simulink model "receiver1"  (R2025a)
settings: Solver=FixedStepAuto  StartTime=0.0  StopTime=10.0  RelTol=1e-3
undefined symbols (not defined in the file): q
libraries: androiduilib x3, dspxfrm3 x2, androidaudiovideolib x1, androidcommunicationlib x1
settings Model: Creator=sahas  LastModifiedBy=sahas
settings OptimizationCC: DefaultParameterBehavior=Inlined  EnhancedBackFolding=on  PassReuseOutputArgsAs=Individual arguments  ZeroExternalMemoryAtStartup=off  ZeroInternalMemoryAtStartup=off  MaxStackSize=64  OptimizeBlockOrder=speed  DifferentSizesBufferReuse=on  OptimizationCustomize=off  EfficientTunableParamExpr=on
settings DebuggingCC: ParameterTunabilityLossMsg=error
settings HardwareCC: ProdBitPerLong=64.0  ProdLargestAtomicInteger=LongLong  ProdLargestAtomicFloat=Double  ProdLongLongMode=on  ProdHWDeviceType=ARM Compatible->ARM Cortex-A (64-bit)  UseEmbeddedCoderFeatures=off
settings SFSimCC: MATLABDynamicMemAlloc=off
settings RTWCC: SystemTargetFile=ert.tlc  HardwareBoard=Android Device (64bit)  TLCOptions="-aInlineSetEventsForThisBaseRateFcn=TLC_FALSE -aSuppressMultiTaskScheduler=TLC_FALSE  -aRateBasedStepFcn=0"  TemplateMakefile=ert_default_tmf  RTWVerbose=off  Toolchain=Android SDK/NDK Tools  Description=Embedded Coder
settings CodeAppCC: ForceParamTrailComments=on  IgnoreCustomStorageClasses=off  OperatorAnnotations=on  SimulinkDataObjDesc=on  SFDataObjDesc=on  InsertBlockDesc=on
settings ERTTargetCC: ExtModeTransport=0.0  ExtModeStaticAlloc=off  ExtModeMexFile=ext_comm  ExtModeIntrfLevel=Level1  SupportNonInlinedSFcns=on

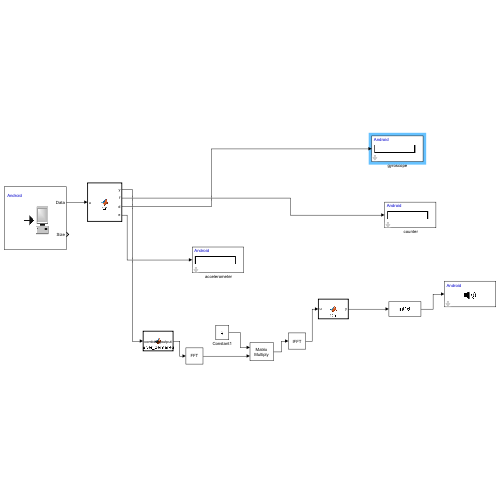
[thumbnail: Simulink's stored preview of the top-level diagram]
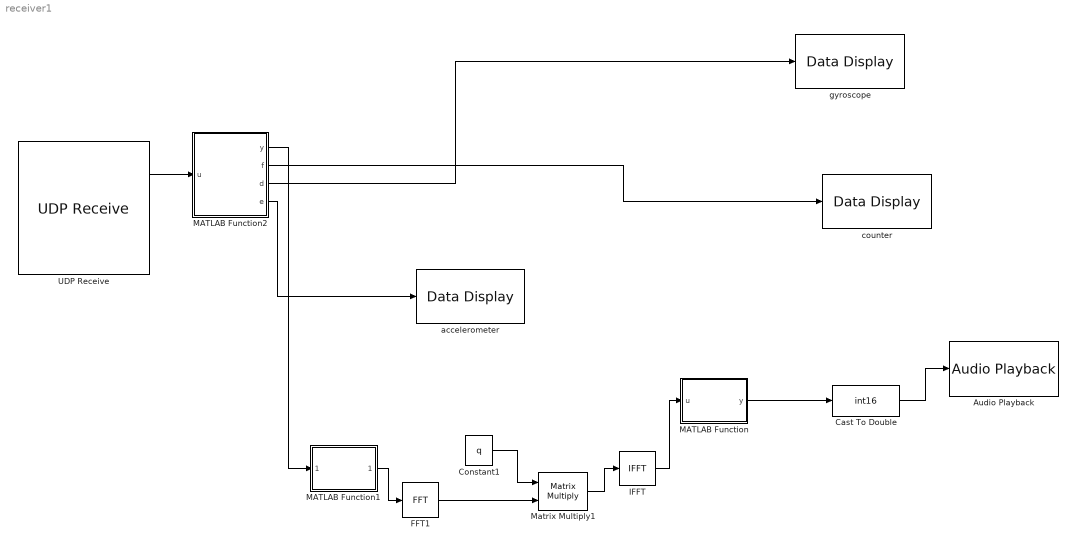
== system receiver1 ==
  " accelerometer" : androiduilib/Data Display  DataDisplayId=receiver1/_accelerometer  Format=Float  Precision=6  SimulateUsing=Code generation  blockPlatform=Android
  " counter" : androiduilib/Data Display  DataDisplayId=receiver1/_counter  Format=Float  Precision=6  SimulateUsing=Code generation  blockPlatform=Android
  Audio Playback : androidaudiovideolib/Audio Playback  SampleFreq=16000  AudioSamplingFreq=16000  SampleTime=0.1  DeviceStr=0  QueueDuration=0  BlockPlatform=Android
  Cast To Double : DataTypeConversion  OutDataTypeStr=int16  SaturateOnIntegerOverflow=off  RndMeth=Floor
  Constant1 : Constant  Value=q  VectorParams1D=off
  FFT1 : dspxfrm3/FFT  FFTImplementation=Auto  CompMethod=Table lookup  TableOpt=NEW  TableOptActive=Speed  BitRevOrder=off  Normalize=off  InheritFFTLength=on  FFTLength=64  WrapInput=on  roundingMode=Ceiling  overflowMode=off  firstCoeffDataTypeStr=Inherit: Same word length as input  firstCoeffLastDataTypeStr=Inherit: Same word length as input  outputMin=[]  outputMax=[]
  IFFT : dspxfrm3/IFFT  FFTImplementation=Auto  CompMethod=Table lookup  TableOpt=NEW  TableOptActive=Speed  BitRevOrder=off  cs_in=off  Normalize=on  InheritFFTLength=on  FFTLength=64  WrapInput=on  mode=Real  outSamplingMode=Sample based  roundingMode=Ceiling  overflowMode=off  firstCoeffDataTypeStr=Inherit: Same word length as input  firstCoeffLastDataTypeStr=Inherit: Same word length as input  outputMin=[]  outputMax=[]
  MATLAB Function : MATLAB Function  TreatAsAtomicUnit=on
  MATLAB Function1 : MATLAB Function  TreatAsAtomicUnit=on
  MATLAB Function2 : MATLAB Function  TreatAsAtomicUnit=on
  Matrix Multiply1 : Product  Multiplication=Matrix(*)
  UDP Receive : androidcommunicationlib/UDP Receive  localURL='0.0.0.0'  localPort=28000  remoteURL='0.0.0.0'  remotePort=-1  recvBufferSize=8192  signalDatatype=double  dims=1031  isVarSize=off  showBlockingTime=off  blockingTime=0  sampletime=0.016  blockPlatform=Android
  gyroscope : androiduilib/Data Display  DataDisplayId=receiver1/gyroscope  Format=Float  Precision=6  SimulateUsing=Code generation  blockPlatform=Android
  wires:
  MATLAB Function1/1(ifft_output) -> FFT1/1
  FFT1/1 -> Matrix Multiply1/2
  Constant1/1 -> Matrix Multiply1/1
  Matrix Multiply1/1 -> IFFT/1
  IFFT/1 -> MATLAB Function/1(u)
  MATLAB Function/1(y) -> Cast To Double/1
  Cast To Double/1 -> Audio Playback/1
  UDP Receive/1 -> MATLAB Function2/1(u)
  MATLAB Function2/1(y) -> MATLAB Function1/1(combined)
  MATLAB Function2/3(d) -> gyroscope/1
  MATLAB Function2/4(e) -> " accelerometer"/1
  MATLAB Function2/2(f) -> " counter"/1

== matlab function receiver1/MATLAB Function1 ==
  data: combined input; ifft_output output
function ifft_output = receiver_deinterleave(combined)
%#codegen

% Convert back to double if needed
combined = double(combined);

N = length(combined)/2;  % number of complex elements

% De-interleave real and imaginary parts
real_flat = combined(1:2:end);
imag_flat = combined(2:2:end);

% Reshape to original 512x2 matrix
real_part = reshape(real_flat, [256,2]);
imag_part = reshape(imag_flat, [256,2]);

% Reconstruct complex IFFT output
ifft_output = real_part + 1j*imag_part;
end

== matlab function receiver1/MATLAB Function ==
  data: u input; y output
function y = fcn(u)

y = real(u);

== matlab function receiver1/MATLAB Function2 ==
  data: u input; y output; f output; d output; e output

function [y,f,d,e]= fcn(u)
f=u(1);
y = u(2:1025);
d=u(1026:1028);
e=u(1029:1031);
